simulink subsystem "Sub_Luces"  (R2023b)
settings: Solver=VariableStepAuto  StartTime=0.0  StopTime=10.0  RelTol=1e-3
libraries: arduinolib x3, simulink x1
settings Model: Creator=Usuario  LastModifiedBy=Pablo

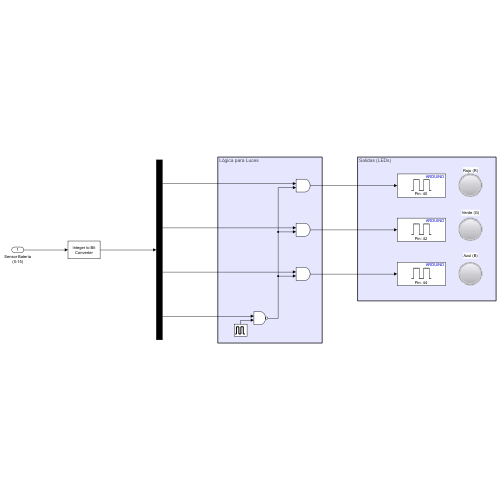
[thumbnail: Simulink's stored preview of the top-level diagram]
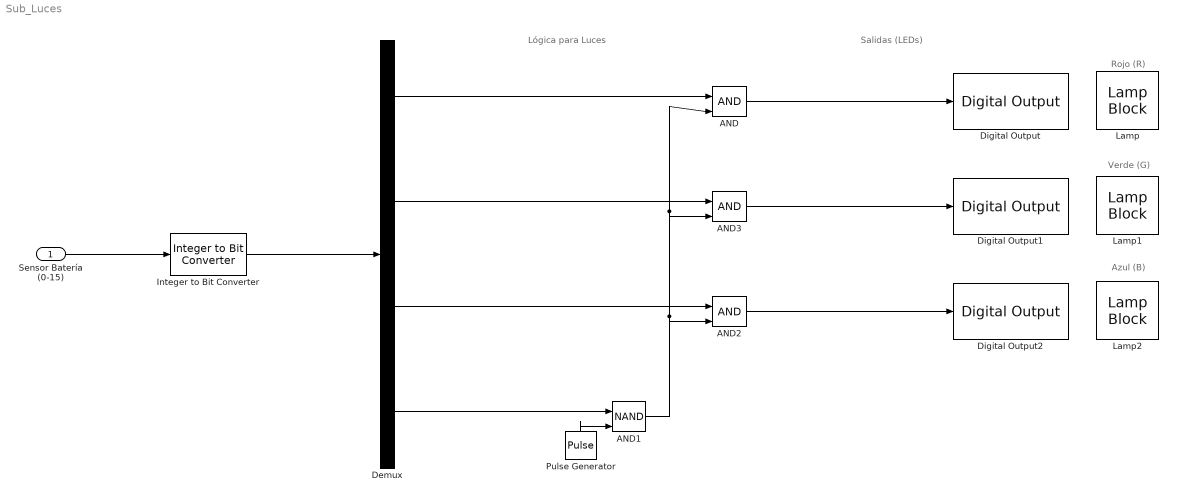
== system Sub_Luces ==
  note: Salidas (LEDs)
  note: Rojo (R)
  note: Lógica para Luces
  note: Verde (G)
  note: Azul (B)
  Sensor Batería (0-15) : Inport
  AND : Logic  IconShape=distinctive  AllPortsSameDT=off  OutDataTypeStr=boolean
  AND1 : Logic  Operator=NAND  IconShape=distinctive  AllPortsSameDT=off  OutDataTypeStr=boolean
  AND2 : Logic  IconShape=distinctive  AllPortsSameDT=off  OutDataTypeStr=boolean
  AND3 : Logic  IconShape=distinctive  AllPortsSameDT=off  OutDataTypeStr=boolean
  Demux : Demux
  Digital Output : arduinolib/Digital Output  pinNumber=40  Direction=output  blockPlatform=arduino
  Digital Output1 : arduinolib/Digital Output  pinNumber=42  Direction=output  blockPlatform=arduino
  Digital Output2 : arduinolib/Digital Output  pinNumber=44  Direction=output  blockPlatform=arduino
  Integer to Bit Converter : simulink/Logic and Bit Operations/Integer to Bit Converter  nbits=4  signedInputValues=Unsigned  bitOrder=MSB first  outDtype=Inherit via internal rule
  Lamp : LampBlock  LabelPosition=Hide
  Lamp1 : LampBlock  LabelPosition=Hide
  Lamp2 : LampBlock  LabelPosition=Hide
  Pulse Generator : DiscretePulseGenerator  PulseType=Time based  Period=1  PulseWidth=50
  wires:
  Sensor Batería (0-15)/1 -> Integer to Bit Converter/1
  Demux/4 -> AND1/1
  Integer to Bit Converter/1 -> Demux/1
  Pulse Generator/1 -> AND1/2
  AND/1 -> Digital Output/1
  AND2/1 -> Digital Output2/1
  Demux/1 -> AND/1
  AND1/1 -> AND2/2, AND3/2, AND/2
  AND3/1 -> Digital Output1/1
  Demux/2 -> AND3/1
  Demux/3 -> AND2/1
